simulink model "QuaternionToAngles"  (R2018a)
settings: Solver=VariableStepAuto  StartTime=0.0  StopTime=10.0  RelTol=1e-3
settings Model: Creator=DEHAEZE  LastModifiedBy=DEHAEZE
settings DataIOCC: SaveOutput=off  SignalLogging=off  DSMLogging=off  SaveTime=off

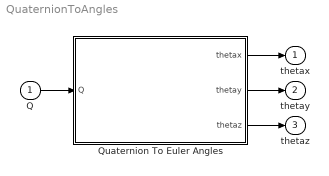
== system QuaternionToAngles ==
  Q : Inport  OutDataTypeStr=double  PortDimensions=4  Interpolate=off
  Quaternion To Euler Angles : MATLAB Function  TreatAsAtomicUnit=on
  thetax : Outport  OutDataTypeStr=double  PortDimensions=1
  thetay : Outport  Port=2  OutDataTypeStr=double  PortDimensions=1
  thetaz : Outport  Port=3  OutDataTypeStr=double  PortDimensions=1
  wires:
  Q/1 -> Quaternion To Euler Angles/1(Q)
  Quaternion To Euler Angles/1(thetax) -> thetax/1
  Quaternion To Euler Angles/2(thetay) -> thetay/1
  Quaternion To Euler Angles/3(thetaz) -> thetaz/1

== matlab function QuaternionToAngles/Quaternion To Euler Angles ==
  data: Q input; thetax output; thetay output; thetaz output
function [thetax, thetay, thetaz] = quaternionToEulerAngles(Q)
thetax = atan2(2*(Q(1)*Q(2) + Q(3)*Q(4)), 1-2*(Q(2)^2+Q(3)^2));
thetay = asin(2*(Q(1)*Q(3)-Q(4)*Q(2)));
thetaz = atan2(2*(Q(1)*Q(4) + Q(2)*Q(3)), 1-2*(Q(3)^2+Q(4)^2));
end
